simulink model "model_sim_CHB5_36_new_temp"  (R2020a)
settings: Solver=FixedStepAuto  StartTime=0.0  StopTime=5  RelTol=1e-3
InitFcn:
  | sysinit
values from neighbouring files (symbols this model uses):
  C = 0.03    [sysinit.m]
  C_f = 0.625e-6    (= 6.25e-07)    [sysinit.m]
  f = 50    [sysinit.m]
  f_switch = 500    [sysinit.m]
  L = 0.004    [sysinit.m]
  L_f = 3e-6    (= 3e-06)    [sysinit.m]
  R = 1.2    [sysinit.m]
  R_f = 1.5    [sysinit.m]
  Rth_h = 7.5e-3    (= 0.0075)    [Device_Parameter.m]
  Rth_h_tau = 0.5    [Device_Parameter.m]
  st = 5e-7    (= 5e-07)    [sysinit.m]
  temp_init = 40    [sysinit.m]
  Ts = 1e-6    (= 1e-06)    [sysinit.m]
  Ts2 = 0.5E-3    (= 0.0005)    [sysinit.m]
  Udc = 2500    [sysinit.m]
undefined symbols (not defined in the file or in its folder): DIODE_204520, DIODE_344520, DIODE_D1031SH, DIODE_D1331SH, IGCT_364520_36, IGCT_364521_36, IGCT_654522_6, magnitude, Ts1
libraries: powerlib x278, powerlib_meascontrol x84, simulink x9
(part 4 of 5)

== system model_sim_CHB5_36_new_temp/Subsystem3/DIODE/DIODE_204520/Subsystem5/Subsystem1 ==
  note: 用于判断D1关断时刻，电流为负时，T3开通就意味着D1关断
  In1 : Inport
  In2 : Inport  Port=2
  Abs1 : Abs
  Add : Sum
  Constant1 : Constant  Value=0
  Constant2 : Constant  Value=0
  Gain1 : Gain  Gain=Udc/DIODE.Vdc
  Gain2 : Gain  Gain=DIODE.Err/DIODE.IFQ
  Gain3 : Gain  Gain=1/Ts2
  Gain4 : Gain
  Logical Operator2 : Logic  Operator=NOT  AllPortsSameDT=off  OutDataTypeStr=boolean
  Logical Operator3 : Logic  AllPortsSameDT=off  OutDataTypeStr=boolean
  Logical Operator4 : Logic  AllPortsSameDT=off  OutDataTypeStr=boolean
  Logical Operator5 : Logic  Operator=NOT  AllPortsSameDT=off  OutDataTypeStr=boolean
  Pulse Generator : DiscretePulseGenerator  PulseType=Time based  Period=Ts2  PulseWidth=5
  Saturation : Saturate  UpperLimit=5500  LowerLimit=0
  Saturation1 : Saturate  UpperLimit=100  LowerLimit=0
  Switch2 : Switch  Criteria=u2 > Threshold
  Switch3 : Switch  Criteria=u2 > Threshold
  Switch4 : Switch  Criteria=u2 > Threshold
  Unit Delay{,1..3} (4 alike) : UnitDelay  SampleTime=Ts1  HasFrameUpgradeWarning=on
  Out1 : Outport  VectorParamsAs1DForOutWhenUnconnected=off
  wires:
  Gain2/1 -> Saturation1/1
  Saturation/1 -> Gain2/1
  Saturation1/1 -> Switch2/1
  Gain4/1 -> Saturation/1
  Unit Delay/1 -> Logical Operator2/1
  Add/1 -> Unit Delay1/1
  In1/1 -> Gain4/1
  Gain3/1 -> Out1/1
  Unit Delay1/1 -> Switch4/1, Switch3/3
  Logical Operator4/1 -> Switch3/2, Switch4/2
  Logical Operator5/1 -> Logical Operator4/2
  Unit Delay3/1 -> Logical Operator5/1
  Unit Delay2/1 -> Switch4/3
  Switch4/1 -> Gain3/1, Unit Delay2/1
  Pulse Generator/1 -> Logical Operator4/1, Unit Delay3/1
  Constant1/1 -> Switch3/1
  Switch3/1 -> Add/2
  Constant2/1 -> Switch2/3
  Logical Operator3/1 -> Switch2/2
  Logical Operator2/1 -> Logical Operator3/2
  In2/1 -> Unit Delay/1, Logical Operator3/1
  Gain1/1 -> Abs1/1
  Switch2/1 -> Gain1/1
  Abs1/1 -> Add/1

== system model_sim_CHB5_36_new_temp/Subsystem3/DIODE/DIODE_204520/Subsystem5/Subsystem2 ==
  note: 器件手册热阻：壳到结
  note: 散热器热阻：水到壳
  In1 : Inport
  In2 : Inport  Port=2
  Add3 : Sum
  Add4 : Sum  Inputs=4
  Add5 : Sum  Inputs=+++
  Constant : Constant  Value=temp_init
  Discrete Filter1 : DiscreteFilter  Numerator=[Ts2/DIODE_344520.Rth_jc1_dou_tau]  Denominator=[1 (Ts2/DIODE_344520.Rth_jc1_dou_tau)-1]  SampleTime=Ts2
  Discrete Filter2 : DiscreteFilter  Numerator=[Ts2/DIODE_344520.Rth_jc2_dou_tau]  Denominator=[1 (Ts2/DIODE_344520.Rth_jc2_dou_tau)-1]  SampleTime=Ts2
  Discrete Filter3 : DiscreteFilter  Numerator=[Ts2/DIODE_344520.Rth_jc3_dou_tau]  Denominator=[1 (Ts2/DIODE_344520.Rth_jc3_dou_tau)-1]  SampleTime=Ts2
  Discrete Filter5 : DiscreteFilter  Numerator=[Ts2/DIODE_344520.Rth_ch_dou_tau]  Denominator=[1 (Ts2/DIODE_344520.Rth_ch_dou_tau)-1]  SampleTime=Ts2
  Discrete Filter9 : DiscreteFilter  Numerator=[Ts2/Rth_h_tau]  Denominator=[1 (Ts2/Rth_h_tau)-1]  SampleTime=Ts2
  Gain1 : Gain  Gain=DIODE_344520.Rth_jc1_dou
  Gain2 : Gain  Gain=DIODE_344520.Rth_jc2_dou
  Gain3 : Gain  Gain=DIODE_344520.Rth_jc3_dou
  Gain5 : Gain  Gain=DIODE_344520.Rth_ch_dou
  Gain9 : Gain  Gain=Rth_h
  Out1 : Outport  VectorParamsAs1DForOutWhenUnconnected=off
  wires:
  Discrete Filter9/1 -> Add5/1
  Gain9/1 -> Discrete Filter9/1
  Add3/1 -> Gain2/1, Gain1/1, Gain9/1, Gain5/1, Gain3/1
  Discrete Filter3/1 -> Add4/4
  Gain3/1 -> Discrete Filter3/1
  Discrete Filter5/1 -> Add4/1
  Gain5/1 -> Discrete Filter5/1
  Discrete Filter1/1 -> Add4/2
  Add5/1 -> Out1/1
  Gain1/1 -> Discrete Filter1/1
  Constant/1 -> Add5/3
  In2/1 -> Add3/2
  Add4/1 -> Add5/2
  Discrete Filter2/1 -> Add4/3
  Gain2/1 -> Discrete Filter2/1
  In1/1 -> Add3/1

== system model_sim_CHB5_36_new_temp/Subsystem3/DIODE/DIODE_204520/Subsystem5/Subsystem29 ==
  note: 用于判断D1关断时刻，电流为负时，T3开通就意味着D1关断
  In1 : Inport
  In2 : Inport  Port=2
  Abs1 : Abs
  Add : Sum
  Constant1 : Constant  Value=0
  Constant2 : Constant  Value=0
  Gain1 : Gain  Gain=Udc/DIODE.Vdc
  Gain2 : Gain  Gain=DIODE.Err/DIODE.IFQ
  Gain3 : Gain  Gain=1/Ts2
  Gain4 : Gain
  Logical Operator2 : Logic  Operator=NOT  AllPortsSameDT=off  OutDataTypeStr=boolean
  Logical Operator3 : Logic  AllPortsSameDT=off  OutDataTypeStr=boolean
  Logical Operator4 : Logic  AllPortsSameDT=off  OutDataTypeStr=boolean
  Logical Operator5 : Logic  Operator=NOT  AllPortsSameDT=off  OutDataTypeStr=boolean
  Pulse Generator : DiscretePulseGenerator  PulseType=Time based  Period=Ts2  PulseWidth=5
  Saturation : Saturate  UpperLimit=5500  LowerLimit=0
  Saturation1 : Saturate  UpperLimit=100  LowerLimit=0
  Switch2 : Switch  Criteria=u2 > Threshold
  Switch3 : Switch  Criteria=u2 > Threshold
  Switch4 : Switch  Criteria=u2 > Threshold
  Unit Delay{,1..3} (4 alike) : UnitDelay  SampleTime=Ts1  HasFrameUpgradeWarning=on
  Out1 : Outport  VectorParamsAs1DForOutWhenUnconnected=off
  wires:
  Gain2/1 -> Saturation1/1
  Saturation/1 -> Gain2/1
  Saturation1/1 -> Switch2/1
  Gain4/1 -> Saturation/1
  Unit Delay/1 -> Logical Operator2/1
  Add/1 -> Unit Delay1/1
  In1/1 -> Gain4/1
  Gain3/1 -> Out1/1
  Unit Delay1/1 -> Switch4/1, Switch3/3
  Logical Operator4/1 -> Switch3/2, Switch4/2
  Logical Operator5/1 -> Logical Operator4/2
  Unit Delay3/1 -> Logical Operator5/1
  Unit Delay2/1 -> Switch4/3
  Switch4/1 -> Gain3/1, Unit Delay2/1
  Pulse Generator/1 -> Logical Operator4/1, Unit Delay3/1
  Constant1/1 -> Switch3/1
  Switch3/1 -> Add/2
  Constant2/1 -> Switch2/3
  Logical Operator3/1 -> Switch2/2
  Logical Operator2/1 -> Logical Operator3/2
  In2/1 -> Unit Delay/1, Logical Operator3/1
  Gain1/1 -> Abs1/1
  Switch2/1 -> Gain1/1
  Abs1/1 -> Add/1

== system model_sim_CHB5_36_new_temp/Subsystem3/DIODE/DIODE_204520/Subsystem5/Subsystem4 ==
  In1 : Inport
  Gain44 : Gain  Gain=DIODE.rF
  Gain45 : Gain  Gain=DIODE.VF0
  Math Function9 : Math  Operator=magnitude^2  SignedPower=on  SaturateOnIntegerOverflow=on
  Mean79 : powerlib_meascontrol/Measurements/Mean  Freq=2000  Vinit=0  Ts=Ts1
  RMS9 : powerlib_meascontrol/Measurements/RMS  TrueRMS=on  Freq=2000  RMSInit=0  Ts=Ts1
  Out1 : Outport
  Out2 : Outport  Port=2
  wires:
  RMS9/1 -> Math Function9/1
  Gain44/1 -> Out1/1
  Mean79/1 -> Gain45/1
  Math Function9/1 -> Gain44/1
  In1/1 -> Mean79/1, RMS9/1
  Gain45/1 -> Out2/1

== system model_sim_CHB5_36_new_temp/Subsystem3/DIODE/DIODE_204520/Subsystem5/Subsystem53 ==
  note: 器件手册热阻：壳到结
  note: 散热器热阻：水到壳
  In1 : Inport
  In2 : Inport  Port=2
  Add3 : Sum
  Add4 : Sum  Inputs=4
  Add5 : Sum  Inputs=+++
  Constant : Constant  Value=temp_init
  Discrete Filter1 : DiscreteFilter  Numerator=[Ts2/DIODE_344520.Rth_jc1_dou_tau]  Denominator=[1 (Ts2/DIODE_344520.Rth_jc1_dou_tau)-1]  SampleTime=Ts2
  Discrete Filter2 : DiscreteFilter  Numerator=[Ts2/DIODE_344520.Rth_jc2_dou_tau]  Denominator=[1 (Ts2/DIODE_344520.Rth_jc2_dou_tau)-1]  SampleTime=Ts2
  Discrete Filter3 : DiscreteFilter  Numerator=[Ts2/DIODE_344520.Rth_jc3_dou_tau]  Denominator=[1 (Ts2/DIODE_344520.Rth_jc3_dou_tau)-1]  SampleTime=Ts2
  Discrete Filter5 : DiscreteFilter  Numerator=[Ts2/DIODE_344520.Rth_ch_dou_tau]  Denominator=[1 (Ts2/DIODE_344520.Rth_ch_dou_tau)-1]  SampleTime=Ts2
  Discrete Filter9 : DiscreteFilter  Numerator=[Ts2/Rth_h_tau]  Denominator=[1 (Ts2/Rth_h_tau)-1]  SampleTime=Ts2
  Gain1 : Gain  Gain=DIODE_344520.Rth_jc1_dou
  Gain2 : Gain  Gain=DIODE_344520.Rth_jc2_dou
  Gain3 : Gain  Gain=DIODE_344520.Rth_jc3_dou
  Gain5 : Gain  Gain=DIODE_344520.Rth_ch_dou
  Gain9 : Gain  Gain=Rth_h
  Out1 : Outport  VectorParamsAs1DForOutWhenUnconnected=off
  wires:
  Discrete Filter9/1 -> Add5/1
  Gain9/1 -> Discrete Filter9/1
  Add3/1 -> Gain2/1, Gain1/1, Gain9/1, Gain5/1, Gain3/1
  Discrete Filter3/1 -> Add4/4
  Gain3/1 -> Discrete Filter3/1
  Discrete Filter5/1 -> Add4/1
  Gain5/1 -> Discrete Filter5/1
  Discrete Filter1/1 -> Add4/2
  Add5/1 -> Out1/1
  Gain1/1 -> Discrete Filter1/1
  Constant/1 -> Add5/3
  In2/1 -> Add3/2
  Add4/1 -> Add5/2
  Discrete Filter2/1 -> Add4/3
  Gain2/1 -> Discrete Filter2/1
  In1/1 -> Add3/1

== system model_sim_CHB5_36_new_temp/Subsystem3/DIODE/DIODE_344520/Subsystem5/Subsystem ==
  In1 : Inport
  Gain44 : Gain  Gain=DIODE.rF
  Gain45 : Gain  Gain=DIODE.VF0
  Math Function9 : Math  Operator=magnitude^2  SignedPower=on  SaturateOnIntegerOverflow=on
  Mean79 : powerlib_meascontrol/Measurements/Mean  Freq=2000  Vinit=0  Ts=Ts
  RMS9 : powerlib_meascontrol/Measurements/RMS  TrueRMS=on  Freq=2000  RMSInit=0  Ts=Ts1
  Out1 : Outport
  Out2 : Outport  Port=2
  wires:
  Gain45/1 -> Out2/1
  In1/1 -> RMS9/1, Mean79/1
  Math Function9/1 -> Gain44/1
  Mean79/1 -> Gain45/1
  Gain44/1 -> Out1/1
  RMS9/1 -> Math Function9/1

== system model_sim_CHB5_36_new_temp/Subsystem3/DIODE/DIODE_344520/Subsystem5/Subsystem1 ==
  note: 用于判断D1关断时刻，电流为负时，T3开通就意味着D1关断
  In1 : Inport
  In2 : Inport  Port=2
  Abs1 : Abs
  Add : Sum
  Constant1 : Constant  Value=0
  Constant2 : Constant  Value=0
  Gain1 : Gain  Gain=Udc/DIODE.Vdc
  Gain2 : Gain  Gain=DIODE.Err/DIODE.IFQ
  Gain3 : Gain  Gain=1/Ts2
  Gain4 : Gain
  Logical Operator2 : Logic  Operator=NOT  AllPortsSameDT=off  OutDataTypeStr=boolean
  Logical Operator3 : Logic  AllPortsSameDT=off  OutDataTypeStr=boolean
  Logical Operator4 : Logic  AllPortsSameDT=off  OutDataTypeStr=boolean
  Logical Operator5 : Logic  Operator=NOT  AllPortsSameDT=off  OutDataTypeStr=boolean
  Pulse Generator : DiscretePulseGenerator  PulseType=Time based  Period=Ts2  PulseWidth=5
  Saturation : Saturate  UpperLimit=5500  LowerLimit=0
  Saturation1 : Saturate  UpperLimit=100  LowerLimit=0
  Switch2 : Switch  Criteria=u2 > Threshold
  Switch3 : Switch  Criteria=u2 > Threshold
  Switch4 : Switch  Criteria=u2 > Threshold
  Unit Delay{,1..3} (4 alike) : UnitDelay  SampleTime=Ts1  HasFrameUpgradeWarning=on
  Out1 : Outport  VectorParamsAs1DForOutWhenUnconnected=off
  wires:
  Abs1/1 -> Add/1
  Switch2/1 -> Gain1/1
  Gain1/1 -> Abs1/1
  In2/1 -> Logical Operator3/1, Unit Delay/1
  Logical Operator2/1 -> Logical Operator3/2
  Logical Operator3/1 -> Switch2/2
  Constant2/1 -> Switch2/3
  Switch3/1 -> Add/2
  Constant1/1 -> Switch3/1
  Pulse Generator/1 -> Unit Delay3/1, Logical Operator4/1
  Switch4/1 -> Unit Delay2/1, Gain3/1
  Unit Delay2/1 -> Switch4/3
  Unit Delay3/1 -> Logical Operator5/1
  Logical Operator5/1 -> Logical Operator4/2
  Logical Operator4/1 -> Switch4/2, Switch3/2
  Unit Delay1/1 -> Switch3/3, Switch4/1
  Gain3/1 -> Out1/1
  In1/1 -> Gain4/1
  Add/1 -> Unit Delay1/1
  Unit Delay/1 -> Logical Operator2/1
  Gain4/1 -> Saturation/1
  Saturation1/1 -> Switch2/1
  Saturation/1 -> Gain2/1
  Gain2/1 -> Saturation1/1

== system model_sim_CHB5_36_new_temp/Subsystem3/DIODE/DIODE_344520/Subsystem5/Subsystem2 ==
  note: 散热器热阻：水到壳
  note: 器件手册热阻：壳到结
  In1 : Inport
  In2 : Inport  Port=2
  Add3 : Sum
  Add4 : Sum  Inputs=4
  Add5 : Sum  Inputs=+++
  Constant : Constant  Value=temp_init
  Discrete Filter1 : DiscreteFilter  Numerator=[Ts2/DIODE_344520.Rth_jc1_dou_tau]  Denominator=[1 (Ts2/DIODE_344520.Rth_jc1_dou_tau)-1]  SampleTime=Ts2
  Discrete Filter2 : DiscreteFilter  Numerator=[Ts2/DIODE_344520.Rth_jc2_dou_tau]  Denominator=[1 (Ts2/DIODE_344520.Rth_jc2_dou_tau)-1]  SampleTime=Ts2
  Discrete Filter3 : DiscreteFilter  Numerator=[Ts2/DIODE_344520.Rth_jc3_dou_tau]  Denominator=[1 (Ts2/DIODE_344520.Rth_jc3_dou_tau)-1]  SampleTime=Ts2
  Discrete Filter5 : DiscreteFilter  Numerator=[Ts2/DIODE_344520.Rth_ch_dou_tau]  Denominator=[1 (Ts2/DIODE_344520.Rth_ch_dou_tau)-1]  SampleTime=Ts2
  Discrete Filter9 : DiscreteFilter  Numerator=[Ts2/Rth_h_tau]  Denominator=[1 (Ts2/Rth_h_tau)-1]  SampleTime=Ts2
  Gain1 : Gain  Gain=DIODE_344520.Rth_jc1_dou
  Gain2 : Gain  Gain=DIODE_344520.Rth_jc2_dou
  Gain3 : Gain  Gain=DIODE_344520.Rth_jc3_dou
  Gain5 : Gain  Gain=DIODE_344520.Rth_ch_dou
  Gain9 : Gain  Gain=Rth_h
  Out1 : Outport  VectorParamsAs1DForOutWhenUnconnected=off
  wires:
  In1/1 -> Add3/1
  Gain2/1 -> Discrete Filter2/1
  Discrete Filter2/1 -> Add4/3
  Add4/1 -> Add5/2
  In2/1 -> Add3/2
  Constant/1 -> Add5/3
  Gain1/1 -> Discrete Filter1/1
  Add5/1 -> Out1/1
  Discrete Filter1/1 -> Add4/2
  Gain5/1 -> Discrete Filter5/1
  Discrete Filter5/1 -> Add4/1
  Gain3/1 -> Discrete Filter3/1
  Discrete Filter3/1 -> Add4/4
  Add3/1 -> Gain3/1, Gain5/1, Gain9/1, Gain1/1, Gain2/1
  Gain9/1 -> Discrete Filter9/1
  Discrete Filter9/1 -> Add5/1

== system model_sim_CHB5_36_new_temp/Subsystem3/DIODE/DIODE_344520/Subsystem5/Subsystem29 ==
  note: 用于判断D1关断时刻，电流为负时，T3开通就意味着D1关断
  In1 : Inport
  In2 : Inport  Port=2
  Abs1 : Abs
  Add : Sum
  Constant1 : Constant  Value=0
  Constant2 : Constant  Value=0
  Gain1 : Gain  Gain=Udc/DIODE.Vdc
  Gain2 : Gain  Gain=DIODE.Err/DIODE.IFQ
  Gain3 : Gain  Gain=1/Ts2
  Gain4 : Gain
  Logical Operator2 : Logic  Operator=NOT  AllPortsSameDT=off  OutDataTypeStr=boolean
  Logical Operator3 : Logic  AllPortsSameDT=off  OutDataTypeStr=boolean
  Logical Operator4 : Logic  AllPortsSameDT=off  OutDataTypeStr=boolean
  Logical Operator5 : Logic  Operator=NOT  AllPortsSameDT=off  OutDataTypeStr=boolean
  Pulse Generator : DiscretePulseGenerator  PulseType=Time based  Period=Ts2  PulseWidth=5
  Saturation : Saturate  UpperLimit=5500  LowerLimit=0
  Saturation1 : Saturate  UpperLimit=100  LowerLimit=0
  Switch2 : Switch  Criteria=u2 > Threshold
  Switch3 : Switch  Criteria=u2 > Threshold
  Switch4 : Switch  Criteria=u2 > Threshold
  Unit Delay{,1..3} (4 alike) : UnitDelay  SampleTime=Ts1  HasFrameUpgradeWarning=on
  Out1 : Outport  VectorParamsAs1DForOutWhenUnconnected=off
  wires:
  Abs1/1 -> Add/1
  Switch2/1 -> Gain1/1
  Gain1/1 -> Abs1/1
  In2/1 -> Logical Operator3/1, Unit Delay/1
  Logical Operator2/1 -> Logical Operator3/2
  Logical Operator3/1 -> Switch2/2
  Constant2/1 -> Switch2/3
  Switch3/1 -> Add/2
  Constant1/1 -> Switch3/1
  Pulse Generator/1 -> Unit Delay3/1, Logical Operator4/1
  Switch4/1 -> Unit Delay2/1, Gain3/1
  Unit Delay2/1 -> Switch4/3
  Unit Delay3/1 -> Logical Operator5/1
  Logical Operator5/1 -> Logical Operator4/2
  Logical Operator4/1 -> Switch4/2, Switch3/2
  Unit Delay1/1 -> Switch3/3, Switch4/1
  Gain3/1 -> Out1/1
  In1/1 -> Gain4/1
  Add/1 -> Unit Delay1/1
  Unit Delay/1 -> Logical Operator2/1
  Gain4/1 -> Saturation/1
  Saturation1/1 -> Switch2/1
  Saturation/1 -> Gain2/1
  Gain2/1 -> Saturation1/1

== system model_sim_CHB5_36_new_temp/Subsystem3/DIODE/DIODE_344520/Subsystem5/Subsystem4 ==
  In1 : Inport
  Gain44 : Gain  Gain=DIODE.rF
  Gain45 : Gain  Gain=DIODE.VF0
  Math Function9 : Math  Operator=magnitude^2  SignedPower=on  SaturateOnIntegerOverflow=on
  Mean79 : powerlib_meascontrol/Measurements/Mean  Freq=2000  Vinit=0  Ts=Ts1
  RMS9 : powerlib_meascontrol/Measurements/RMS  TrueRMS=on  Freq=2000  RMSInit=0  Ts=Ts1
  Out1 : Outport
  Out2 : Outport  Port=2
  wires:
  Gain45/1 -> Out2/1
  In1/1 -> RMS9/1, Mean79/1
  Math Function9/1 -> Gain44/1
  Mean79/1 -> Gain45/1
  Gain44/1 -> Out1/1
  RMS9/1 -> Math Function9/1

== system model_sim_CHB5_36_new_temp/Subsystem3/DIODE/DIODE_344520/Subsystem5/Subsystem53 ==
  note: 散热器热阻：水到壳
  note: 器件手册热阻：壳到结
  In1 : Inport
  In2 : Inport  Port=2
  Add3 : Sum
  Add4 : Sum  Inputs=4
  Add5 : Sum  Inputs=+++
  Constant : Constant  Value=temp_init
  Discrete Filter1 : DiscreteFilter  Numerator=[Ts2/DIODE_344520.Rth_jc1_dou_tau]  Denominator=[1 (Ts2/DIODE_344520.Rth_jc1_dou_tau)-1]  SampleTime=Ts2
  Discrete Filter2 : DiscreteFilter  Numerator=[Ts2/DIODE_344520.Rth_jc2_dou_tau]  Denominator=[1 (Ts2/DIODE_344520.Rth_jc2_dou_tau)-1]  SampleTime=Ts2
  Discrete Filter3 : DiscreteFilter  Numerator=[Ts2/DIODE_344520.Rth_jc3_dou_tau]  Denominator=[1 (Ts2/DIODE_344520.Rth_jc3_dou_tau)-1]  SampleTime=Ts2
  Discrete Filter5 : DiscreteFilter  Numerator=[Ts2/DIODE_344520.Rth_ch_dou_tau]  Denominator=[1 (Ts2/DIODE_344520.Rth_ch_dou_tau)-1]  SampleTime=Ts2
  Discrete Filter9 : DiscreteFilter  Numerator=[Ts2/Rth_h_tau]  Denominator=[1 (Ts2/Rth_h_tau)-1]  SampleTime=Ts2
  Gain1 : Gain  Gain=DIODE_344520.Rth_jc1_dou
  Gain2 : Gain  Gain=DIODE_344520.Rth_jc2_dou
  Gain3 : Gain  Gain=DIODE_344520.Rth_jc3_dou
  Gain5 : Gain  Gain=DIODE_344520.Rth_ch_dou
  Gain9 : Gain  Gain=Rth_h
  Out1 : Outport  VectorParamsAs1DForOutWhenUnconnected=off
  wires:
  In1/1 -> Add3/1
  Gain2/1 -> Discrete Filter2/1
  Discrete Filter2/1 -> Add4/3
  Add4/1 -> Add5/2
  In2/1 -> Add3/2
  Constant/1 -> Add5/3
  Gain1/1 -> Discrete Filter1/1
  Add5/1 -> Out1/1
  Discrete Filter1/1 -> Add4/2
  Gain5/1 -> Discrete Filter5/1
  Discrete Filter5/1 -> Add4/1
  Gain3/1 -> Discrete Filter3/1
  Discrete Filter3/1 -> Add4/4
  Add3/1 -> Gain3/1, Gain5/1, Gain9/1, Gain1/1, Gain2/1
  Gain9/1 -> Discrete Filter9/1
  Discrete Filter9/1 -> Add5/1

== system model_sim_CHB5_36_new_temp/Subsystem3/DIODE/DIODE_D1031SH/Subsystem5/Subsystem ==
  In1 : Inport
  Gain44 : Gain  Gain=DIODE.rF
  Gain45 : Gain  Gain=DIODE.VF0
  Math Function9 : Math  Operator=magnitude^2  SignedPower=on  SaturateOnIntegerOverflow=on
  Mean79 : powerlib_meascontrol/Measurements/Mean  Freq=2000  Vinit=0  Ts=Ts1
  RMS9 : powerlib_meascontrol/Measurements/RMS  TrueRMS=on  Freq=2000  RMSInit=0  Ts=Ts1
  Out1 : Outport
  Out2 : Outport  Port=2
  wires:
  RMS9/1 -> Math Function9/1
  Gain44/1 -> Out1/1
  Mean79/1 -> Gain45/1
  Math Function9/1 -> Gain44/1
  In1/1 -> Mean79/1, RMS9/1
  Gain45/1 -> Out2/1

== system model_sim_CHB5_36_new_temp/Subsystem3/DIODE/DIODE_D1031SH/Subsystem5/Subsystem1 ==
  note: 用于判断D1关断时刻，电流为负时，T3开通就意味着D1关断
  In1 : Inport
  In2 : Inport  Port=2
  Abs1 : Abs
  Add : Sum
  Constant1 : Constant  Value=0
  Constant2 : Constant  Value=0
  Gain1 : Gain  Gain=Udc/DIODE.Vdc
  Gain2 : Gain  Gain=DIODE.Err/DIODE.IFQ
  Gain3 : Gain  Gain=1/Ts2
  Gain4 : Gain
  Logical Operator2 : Logic  Operator=NOT  AllPortsSameDT=off  OutDataTypeStr=boolean
  Logical Operator3 : Logic  AllPortsSameDT=off  OutDataTypeStr=boolean
  Logical Operator4 : Logic  AllPortsSameDT=off  OutDataTypeStr=boolean
  Logical Operator5 : Logic  Operator=NOT  AllPortsSameDT=off  OutDataTypeStr=boolean
  Pulse Generator : DiscretePulseGenerator  PulseType=Time based  Period=Ts2  PulseWidth=5
  Saturation : Saturate  UpperLimit=5500  LowerLimit=0
  Saturation1 : Saturate  UpperLimit=100  LowerLimit=0
  Switch2 : Switch  Criteria=u2 > Threshold
  Switch3 : Switch  Criteria=u2 > Threshold
  Switch4 : Switch  Criteria=u2 > Threshold
  Unit Delay{,1..3} (4 alike) : UnitDelay  SampleTime=Ts1  HasFrameUpgradeWarning=on
  Out1 : Outport  VectorParamsAs1DForOutWhenUnconnected=off
  wires:
  Gain2/1 -> Saturation1/1
  Saturation/1 -> Gain2/1
  Saturation1/1 -> Switch2/1
  Gain4/1 -> Saturation/1
  Unit Delay/1 -> Logical Operator2/1
  Add/1 -> Unit Delay1/1
  In1/1 -> Gain4/1
  Gain3/1 -> Out1/1
  Unit Delay1/1 -> Switch4/1, Switch3/3
  Logical Operator4/1 -> Switch3/2, Switch4/2
  Logical Operator5/1 -> Logical Operator4/2
  Unit Delay3/1 -> Logical Operator5/1
  Unit Delay2/1 -> Switch4/3
  Switch4/1 -> Gain3/1, Unit Delay2/1
  Pulse Generator/1 -> Logical Operator4/1, Unit Delay3/1
  Constant1/1 -> Switch3/1
  Switch3/1 -> Add/2
  Constant2/1 -> Switch2/3
  Logical Operator3/1 -> Switch2/2
  Logical Operator2/1 -> Logical Operator3/2
  In2/1 -> Unit Delay/1, Logical Operator3/1
  Gain1/1 -> Abs1/1
  Switch2/1 -> Gain1/1
  Abs1/1 -> Add/1

== system model_sim_CHB5_36_new_temp/Subsystem3/DIODE/DIODE_D1031SH/Subsystem5/Subsystem2 ==
  note: 器件手册热阻：壳到结
  note: 散热器热阻：水到壳
  In1 : Inport
  In2 : Inport  Port=2
  Add3 : Sum
  Add4 : Sum  Inputs=4
  Add5 : Sum  Inputs=+++
  Constant : Constant  Value=temp_init
  Discrete Filter1 : DiscreteFilter  Numerator=[Ts2/DIODE_344520.Rth_jc1_dou_tau]  Denominator=[1 (Ts2/DIODE_344520.Rth_jc1_dou_tau)-1]  SampleTime=Ts2
  Discrete Filter2 : DiscreteFilter  Numerator=[Ts2/DIODE_344520.Rth_jc2_dou_tau]  Denominator=[1 (Ts2/DIODE_344520.Rth_jc2_dou_tau)-1]  SampleTime=Ts2
  Discrete Filter3 : DiscreteFilter  Numerator=[Ts2/DIODE_344520.Rth_jc3_dou_tau]  Denominator=[1 (Ts2/DIODE_344520.Rth_jc3_dou_tau)-1]  SampleTime=Ts2
  Discrete Filter5 : DiscreteFilter  Numerator=[Ts2/DIODE_344520.Rth_ch_dou_tau]  Denominator=[1 (Ts2/DIODE_344520.Rth_ch_dou_tau)-1]  SampleTime=Ts2
  Discrete Filter9 : DiscreteFilter  Numerator=[Ts2/Rth_h_tau]  Denominator=[1 (Ts2/Rth_h_tau)-1]  SampleTime=Ts2
  Gain1 : Gain  Gain=DIODE_344520.Rth_jc1_dou
  Gain2 : Gain  Gain=DIODE_344520.Rth_jc2_dou
  Gain3 : Gain  Gain=DIODE_344520.Rth_jc3_dou
  Gain5 : Gain  Gain=DIODE_344520.Rth_ch_dou
  Gain9 : Gain  Gain=Rth_h
  Out1 : Outport  VectorParamsAs1DForOutWhenUnconnected=off
  wires:
  Discrete Filter9/1 -> Add5/1
  Gain9/1 -> Discrete Filter9/1
  Add3/1 -> Gain2/1, Gain1/1, Gain9/1, Gain5/1, Gain3/1
  Discrete Filter3/1 -> Add4/4
  Gain3/1 -> Discrete Filter3/1
  Discrete Filter5/1 -> Add4/1
  Gain5/1 -> Discrete Filter5/1
  Discrete Filter1/1 -> Add4/2
  Add5/1 -> Out1/1
  Gain1/1 -> Discrete Filter1/1
  Constant/1 -> Add5/3
  In2/1 -> Add3/2
  Add4/1 -> Add5/2
  Discrete Filter2/1 -> Add4/3
  Gain2/1 -> Discrete Filter2/1
  In1/1 -> Add3/1

== system model_sim_CHB5_36_new_temp/Subsystem3/DIODE/DIODE_D1031SH/Subsystem5/Subsystem29 ==
  note: 用于判断D1关断时刻，电流为负时，T3开通就意味着D1关断
  In1 : Inport
  In2 : Inport  Port=2
  Abs1 : Abs
  Add : Sum
  Constant1 : Constant  Value=0
  Constant2 : Constant  Value=0
  Gain1 : Gain  Gain=Udc/DIODE.Vdc
  Gain2 : Gain  Gain=DIODE.Err/DIODE.IFQ
  Gain3 : Gain  Gain=1/Ts2
  Gain4 : Gain
  Logical Operator2 : Logic  Operator=NOT  AllPortsSameDT=off  OutDataTypeStr=boolean
  Logical Operator3 : Logic  AllPortsSameDT=off  OutDataTypeStr=boolean
  Logical Operator4 : Logic  AllPortsSameDT=off  OutDataTypeStr=boolean
  Logical Operator5 : Logic  Operator=NOT  AllPortsSameDT=off  OutDataTypeStr=boolean
  Pulse Generator : DiscretePulseGenerator  PulseType=Time based  Period=Ts2  PulseWidth=5
  Saturation : Saturate  UpperLimit=5500  LowerLimit=0
  Saturation1 : Saturate  UpperLimit=100  LowerLimit=0
  Switch2 : Switch  Criteria=u2 > Threshold
  Switch3 : Switch  Criteria=u2 > Threshold
  Switch4 : Switch  Criteria=u2 > Threshold
  Unit Delay{,1..3} (4 alike) : UnitDelay  SampleTime=Ts1  HasFrameUpgradeWarning=on
  Out1 : Outport  VectorParamsAs1DForOutWhenUnconnected=off
  wires:
  Gain2/1 -> Saturation1/1
  Saturation/1 -> Gain2/1
  Saturation1/1 -> Switch2/1
  Gain4/1 -> Saturation/1
  Unit Delay/1 -> Logical Operator2/1
  Add/1 -> Unit Delay1/1
  In1/1 -> Gain4/1
  Gain3/1 -> Out1/1
  Unit Delay1/1 -> Switch4/1, Switch3/3
  Logical Operator4/1 -> Switch3/2, Switch4/2
  Logical Operator5/1 -> Logical Operator4/2
  Unit Delay3/1 -> Logical Operator5/1
  Unit Delay2/1 -> Switch4/3
  Switch4/1 -> Gain3/1, Unit Delay2/1
  Pulse Generator/1 -> Logical Operator4/1, Unit Delay3/1
  Constant1/1 -> Switch3/1
  Switch3/1 -> Add/2
  Constant2/1 -> Switch2/3
  Logical Operator3/1 -> Switch2/2
  Logical Operator2/1 -> Logical Operator3/2
  In2/1 -> Unit Delay/1, Logical Operator3/1
  Gain1/1 -> Abs1/1
  Switch2/1 -> Gain1/1
  Abs1/1 -> Add/1

== system model_sim_CHB5_36_new_temp/Subsystem3/DIODE/DIODE_D1031SH/Subsystem5/Subsystem4 ==
  In1 : Inport
  Gain44 : Gain  Gain=DIODE.rF
  Gain45 : Gain  Gain=DIODE.VF0
  Math Function9 : Math  Operator=magnitude^2  SignedPower=on  SaturateOnIntegerOverflow=on
  Mean79 : powerlib_meascontrol/Measurements/Mean  Freq=2000  Vinit=0  Ts=Ts1
  RMS9 : powerlib_meascontrol/Measurements/RMS  TrueRMS=on  Freq=2000  RMSInit=0  Ts=Ts1
  Out1 : Outport
  Out2 : Outport  Port=2
  wires:
  RMS9/1 -> Math Function9/1
  Gain44/1 -> Out1/1
  Mean79/1 -> Gain45/1
  Math Function9/1 -> Gain44/1
  In1/1 -> Mean79/1, RMS9/1
  Gain45/1 -> Out2/1

== system model_sim_CHB5_36_new_temp/Subsystem3/DIODE/DIODE_D1031SH/Subsystem5/Subsystem53 ==
  note: 器件手册热阻：壳到结
  note: 散热器热阻：水到壳
  In1 : Inport
  In2 : Inport  Port=2
  Add3 : Sum
  Add4 : Sum  Inputs=4
  Add5 : Sum  Inputs=+++
  Constant : Constant  Value=temp_init
  Discrete Filter1 : DiscreteFilter  Numerator=[Ts2/DIODE_344520.Rth_jc1_dou_tau]  Denominator=[1 (Ts2/DIODE_344520.Rth_jc1_dou_tau)-1]  SampleTime=Ts2
  Discrete Filter2 : DiscreteFilter  Numerator=[Ts2/DIODE_344520.Rth_jc2_dou_tau]  Denominator=[1 (Ts2/DIODE_344520.Rth_jc2_dou_tau)-1]  SampleTime=Ts2
  Discrete Filter3 : DiscreteFilter  Numerator=[Ts2/DIODE_344520.Rth_jc3_dou_tau]  Denominator=[1 (Ts2/DIODE_344520.Rth_jc3_dou_tau)-1]  SampleTime=Ts2
  Discrete Filter5 : DiscreteFilter  Numerator=[Ts2/DIODE_344520.Rth_ch_dou_tau]  Denominator=[1 (Ts2/DIODE_344520.Rth_ch_dou_tau)-1]  SampleTime=Ts2
  Discrete Filter9 : DiscreteFilter  Numerator=[Ts2/Rth_h_tau]  Denominator=[1 (Ts2/Rth_h_tau)-1]  SampleTime=Ts2
  Gain1 : Gain  Gain=DIODE_344520.Rth_jc1_dou
  Gain2 : Gain  Gain=DIODE_344520.Rth_jc2_dou
  Gain3 : Gain  Gain=DIODE_344520.Rth_jc3_dou
  Gain5 : Gain  Gain=DIODE_344520.Rth_ch_dou
  Gain9 : Gain  Gain=Rth_h
  Out1 : Outport  VectorParamsAs1DForOutWhenUnconnected=off
  wires:
  Discrete Filter9/1 -> Add5/1
  Gain9/1 -> Discrete Filter9/1
  Add3/1 -> Gain2/1, Gain1/1, Gain9/1, Gain5/1, Gain3/1
  Discrete Filter3/1 -> Add4/4
  Gain3/1 -> Discrete Filter3/1
  Discrete Filter5/1 -> Add4/1
  Gain5/1 -> Discrete Filter5/1
  Discrete Filter1/1 -> Add4/2
  Add5/1 -> Out1/1
  Gain1/1 -> Discrete Filter1/1
  Constant/1 -> Add5/3
  In2/1 -> Add3/2
  Add4/1 -> Add5/2
  Discrete Filter2/1 -> Add4/3
  Gain2/1 -> Discrete Filter2/1
  In1/1 -> Add3/1

== system model_sim_CHB5_36_new_temp/Subsystem3/DIODE/DIODE_D1331SH/Subsystem5/Subsystem ==
  In1 : Inport
  Gain44 : Gain  Gain=DIODE.rF
  Gain45 : Gain  Gain=DIODE.VF0
  Math Function9 : Math  Operator=magnitude^2  SignedPower=on  SaturateOnIntegerOverflow=on
  Mean79 : powerlib_meascontrol/Measurements/Mean  Freq=2000  Vinit=0  Ts=Ts1
  RMS9 : powerlib_meascontrol/Measurements/RMS  TrueRMS=on  Freq=2000  RMSInit=0  Ts=Ts1
  Out1 : Outport
  Out2 : Outport  Port=2
  wires:
  Gain45/1 -> Out2/1
  In1/1 -> RMS9/1, Mean79/1
  Math Function9/1 -> Gain44/1
  Mean79/1 -> Gain45/1
  Gain44/1 -> Out1/1
  RMS9/1 -> Math Function9/1

== system model_sim_CHB5_36_new_temp/Subsystem3/DIODE/DIODE_D1331SH/Subsystem5/Subsystem1 ==
  note: 用于判断D1关断时刻，电流为负时，T3开通就意味着D1关断
  In1 : Inport
  In2 : Inport  Port=2
  Abs1 : Abs
  Add : Sum
  Constant1 : Constant  Value=0
  Constant2 : Constant  Value=0
  Gain1 : Gain  Gain=Udc/DIODE.Vdc
  Gain2 : Gain  Gain=DIODE.Err/DIODE.IFQ
  Gain3 : Gain  Gain=1/Ts2
  Gain4 : Gain
  Logical Operator2 : Logic  Operator=NOT  AllPortsSameDT=off  OutDataTypeStr=boolean
  Logical Operator3 : Logic  AllPortsSameDT=off  OutDataTypeStr=boolean
  Logical Operator4 : Logic  AllPortsSameDT=off  OutDataTypeStr=boolean
  Logical Operator5 : Logic  Operator=NOT  AllPortsSameDT=off  OutDataTypeStr=boolean
  Pulse Generator : DiscretePulseGenerator  PulseType=Time based  Period=Ts2  PulseWidth=5
  Saturation : Saturate  UpperLimit=5500  LowerLimit=0
  Saturation1 : Saturate  UpperLimit=100  LowerLimit=0
  Switch2 : Switch  Criteria=u2 > Threshold
  Switch3 : Switch  Criteria=u2 > Threshold
  Switch4 : Switch  Criteria=u2 > Threshold
  Unit Delay{,1..3} (4 alike) : UnitDelay  SampleTime=Ts1  HasFrameUpgradeWarning=on
  Out1 : Outport  VectorParamsAs1DForOutWhenUnconnected=off
  wires:
  Abs1/1 -> Add/1
  Switch2/1 -> Gain1/1
  Gain1/1 -> Abs1/1
  In2/1 -> Logical Operator3/1, Unit Delay/1
  Logical Operator2/1 -> Logical Operator3/2
  Logical Operator3/1 -> Switch2/2
  Constant2/1 -> Switch2/3
  Switch3/1 -> Add/2
  Constant1/1 -> Switch3/1
  Pulse Generator/1 -> Unit Delay3/1, Logical Operator4/1
  Switch4/1 -> Unit Delay2/1, Gain3/1
  Unit Delay2/1 -> Switch4/3
  Unit Delay3/1 -> Logical Operator5/1
  Logical Operator5/1 -> Logical Operator4/2
  Logical Operator4/1 -> Switch4/2, Switch3/2
  Unit Delay1/1 -> Switch3/3, Switch4/1
  Gain3/1 -> Out1/1
  In1/1 -> Gain4/1
  Add/1 -> Unit Delay1/1
  Unit Delay/1 -> Logical Operator2/1
  Gain4/1 -> Saturation/1
  Saturation1/1 -> Switch2/1
  Saturation/1 -> Gain2/1
  Gain2/1 -> Saturation1/1

== system model_sim_CHB5_36_new_temp/Subsystem3/DIODE/DIODE_D1331SH/Subsystem5/Subsystem2 ==
  note: 散热器热阻：水到壳
  note: 器件手册热阻：壳到结
  In1 : Inport
  In2 : Inport  Port=2
  Add3 : Sum
  Add4 : Sum  Inputs=4
  Add5 : Sum  Inputs=+++
  Constant : Constant  Value=temp_init
  Discrete Filter1 : DiscreteFilter  Numerator=[Ts2/DIODE_344520.Rth_jc1_dou_tau]  Denominator=[1 (Ts2/DIODE_344520.Rth_jc1_dou_tau)-1]  SampleTime=Ts2
  Discrete Filter2 : DiscreteFilter  Numerator=[Ts2/DIODE_344520.Rth_jc2_dou_tau]  Denominator=[1 (Ts2/DIODE_344520.Rth_jc2_dou_tau)-1]  SampleTime=Ts2
  Discrete Filter3 : DiscreteFilter  Numerator=[Ts2/DIODE_344520.Rth_jc3_dou_tau]  Denominator=[1 (Ts2/DIODE_344520.Rth_jc3_dou_tau)-1]  SampleTime=Ts2
  Discrete Filter5 : DiscreteFilter  Numerator=[Ts2/DIODE_344520.Rth_ch_dou_tau]  Denominator=[1 (Ts2/DIODE_344520.Rth_ch_dou_tau)-1]  SampleTime=Ts2
  Discrete Filter9 : DiscreteFilter  Numerator=[Ts2/Rth_h_tau]  Denominator=[1 (Ts2/Rth_h_tau)-1]  SampleTime=Ts2
  Gain1 : Gain  Gain=DIODE_344520.Rth_jc1_dou
  Gain2 : Gain  Gain=DIODE_344520.Rth_jc2_dou
  Gain3 : Gain  Gain=DIODE_344520.Rth_jc3_dou
  Gain5 : Gain  Gain=DIODE_344520.Rth_ch_dou
  Gain9 : Gain  Gain=Rth_h
  Out1 : Outport  VectorParamsAs1DForOutWhenUnconnected=off
  wires:
  In1/1 -> Add3/1
  Gain2/1 -> Discrete Filter2/1
  Discrete Filter2/1 -> Add4/3
  Add4/1 -> Add5/2
  In2/1 -> Add3/2
  Constant/1 -> Add5/3
  Gain1/1 -> Discrete Filter1/1
  Add5/1 -> Out1/1
  Discrete Filter1/1 -> Add4/2
  Gain5/1 -> Discrete Filter5/1
  Discrete Filter5/1 -> Add4/1
  Gain3/1 -> Discrete Filter3/1
  Discrete Filter3/1 -> Add4/4
  Add3/1 -> Gain3/1, Gain5/1, Gain9/1, Gain1/1, Gain2/1
  Gain9/1 -> Discrete Filter9/1
  Discrete Filter9/1 -> Add5/1

== system model_sim_CHB5_36_new_temp/Subsystem3/DIODE/DIODE_D1331SH/Subsystem5/Subsystem29 ==
  note: 用于判断D1关断时刻，电流为负时，T3开通就意味着D1关断
  In1 : Inport
  In2 : Inport  Port=2
  Abs1 : Abs
  Add : Sum
  Constant1 : Constant  Value=0
  Constant2 : Constant  Value=0
  Gain1 : Gain  Gain=Udc/DIODE.Vdc
  Gain2 : Gain  Gain=DIODE.Err/DIODE.IFQ
  Gain3 : Gain  Gain=1/Ts2
  Gain4 : Gain
  Logical Operator2 : Logic  Operator=NOT  AllPortsSameDT=off  OutDataTypeStr=boolean
  Logical Operator3 : Logic  AllPortsSameDT=off  OutDataTypeStr=boolean
  Logical Operator4 : Logic  AllPortsSameDT=off  OutDataTypeStr=boolean
  Logical Operator5 : Logic  Operator=NOT  AllPortsSameDT=off  OutDataTypeStr=boolean
  Pulse Generator : DiscretePulseGenerator  PulseType=Time based  Period=Ts2  PulseWidth=5
  Saturation : Saturate  UpperLimit=5500  LowerLimit=0
  Saturation1 : Saturate  UpperLimit=100  LowerLimit=0
  Switch2 : Switch  Criteria=u2 > Threshold
  Switch3 : Switch  Criteria=u2 > Threshold
  Switch4 : Switch  Criteria=u2 > Threshold
  Unit Delay{,1..3} (4 alike) : UnitDelay  SampleTime=Ts1  HasFrameUpgradeWarning=on
  Out1 : Outport  VectorParamsAs1DForOutWhenUnconnected=off
  wires:
  Abs1/1 -> Add/1
  Switch2/1 -> Gain1/1
  Gain1/1 -> Abs1/1
  In2/1 -> Logical Operator3/1, Unit Delay/1
  Logical Operator2/1 -> Logical Operator3/2
  Logical Operator3/1 -> Switch2/2
  Constant2/1 -> Switch2/3
  Switch3/1 -> Add/2
  Constant1/1 -> Switch3/1
  Pulse Generator/1 -> Unit Delay3/1, Logical Operator4/1
  Switch4/1 -> Unit Delay2/1, Gain3/1
  Unit Delay2/1 -> Switch4/3
  Unit Delay3/1 -> Logical Operator5/1
  Logical Operator5/1 -> Logical Operator4/2
  Logical Operator4/1 -> Switch4/2, Switch3/2
  Unit Delay1/1 -> Switch3/3, Switch4/1
  Gain3/1 -> Out1/1
  In1/1 -> Gain4/1
  Add/1 -> Unit Delay1/1
  Unit Delay/1 -> Logical Operator2/1
  Gain4/1 -> Saturation/1
  Saturation1/1 -> Switch2/1
  Saturation/1 -> Gain2/1
  Gain2/1 -> Saturation1/1

== system model_sim_CHB5_36_new_temp/Subsystem3/DIODE/DIODE_D1331SH/Subsystem5/Subsystem4 ==
  In1 : Inport
  Gain44 : Gain  Gain=DIODE.rF
  Gain45 : Gain  Gain=DIODE.VF0
  Math Function9 : Math  Operator=magnitude^2  SignedPower=on  SaturateOnIntegerOverflow=on
  Mean79 : powerlib_meascontrol/Measurements/Mean  Freq=2000  Vinit=0  Ts=Ts1
  RMS9 : powerlib_meascontrol/Measurements/RMS  TrueRMS=on  Freq=2000  RMSInit=0  Ts=Ts1
  Out1 : Outport
  Out2 : Outport  Port=2
  wires:
  Gain45/1 -> Out2/1
  In1/1 -> RMS9/1, Mean79/1
  Math Function9/1 -> Gain44/1
  Mean79/1 -> Gain45/1
  Gain44/1 -> Out1/1
  RMS9/1 -> Math Function9/1

== system model_sim_CHB5_36_new_temp/Subsystem3/DIODE/DIODE_D1331SH/Subsystem5/Subsystem53 ==
  note: 散热器热阻：水到壳
  note: 器件手册热阻：壳到结
  In1 : Inport
  In2 : Inport  Port=2
  Add3 : Sum
  Add4 : Sum  Inputs=4
  Add5 : Sum  Inputs=+++
  Constant : Constant  Value=temp_init
  Discrete Filter1 : DiscreteFilter  Numerator=[Ts2/DIODE_344520.Rth_jc1_dou_tau]  Denominator=[1 (Ts2/DIODE_344520.Rth_jc1_dou_tau)-1]  SampleTime=Ts2
  Discrete Filter2 : DiscreteFilter  Numerator=[Ts2/DIODE_344520.Rth_jc2_dou_tau]  Denominator=[1 (Ts2/DIODE_344520.Rth_jc2_dou_tau)-1]  SampleTime=Ts2
  Discrete Filter3 : DiscreteFilter  Numerator=[Ts2/DIODE_344520.Rth_jc3_dou_tau]  Denominator=[1 (Ts2/DIODE_344520.Rth_jc3_dou_tau)-1]  SampleTime=Ts2
  Discrete Filter5 : DiscreteFilter  Numerator=[Ts2/DIODE_344520.Rth_ch_dou_tau]  Denominator=[1 (Ts2/DIODE_344520.Rth_ch_dou_tau)-1]  SampleTime=Ts2
  Discrete Filter9 : DiscreteFilter  Numerator=[Ts2/Rth_h_tau]  Denominator=[1 (Ts2/Rth_h_tau)-1]  SampleTime=Ts2
  Gain1 : Gain  Gain=DIODE_344520.Rth_jc1_dou
  Gain2 : Gain  Gain=DIODE_344520.Rth_jc2_dou
  Gain3 : Gain  Gain=DIODE_344520.Rth_jc3_dou
  Gain5 : Gain  Gain=DIODE_344520.Rth_ch_dou
  Gain9 : Gain  Gain=Rth_h
  Out1 : Outport  VectorParamsAs1DForOutWhenUnconnected=off
  wires:
  In1/1 -> Add3/1
  Gain2/1 -> Discrete Filter2/1
  Discrete Filter2/1 -> Add4/3
  Add4/1 -> Add5/2
  In2/1 -> Add3/2
  Constant/1 -> Add5/3
  Gain1/1 -> Discrete Filter1/1
  Add5/1 -> Out1/1
  Discrete Filter1/1 -> Add4/2
  Gain5/1 -> Discrete Filter5/1
  Discrete Filter5/1 -> Add4/1
  Gain3/1 -> Discrete Filter3/1
  Discrete Filter3/1 -> Add4/4
  Add3/1 -> Gain3/1, Gain5/1, Gain9/1, Gain1/1, Gain2/1
  Gain9/1 -> Discrete Filter9/1
  Discrete Filter9/1 -> Add5/1

== system model_sim_CHB5_36_new_temp/Subsystem3/IGCT/IGCT_364520_36/MAIN/Subsystem3 ==
  i : Inport
  pwm : Inport  Port=2
  Abs1 : Abs
  Add : Sum
  Constant1 : Constant  Value=0
  Constant2 : Constant  Value=0
  Gain1 : Gain  Gain=Udc/IGCT.Vdc
  Gain2 : Gain  Gain=IGCT.Eon/IGCT.IT*Udc/IGCT.Vdc
  Gain3 : Gain  Gain=1/Ts2
  Gain4 : Gain
  Logical Operator : Logic  AllPortsSameDT=off  OutDataTypeStr=boolean
  Logical Operator1 : Logic  Operator=NOT  AllPortsSameDT=off  OutDataTypeStr=boolean
  Logical Operator2 : Logic  Operator=NOT  AllPortsSameDT=off  OutDataTypeStr=boolean
  Logical Operator3 : Logic  AllPortsSameDT=off  OutDataTypeStr=boolean
  Logical Operator4 : Logic  AllPortsSameDT=off  OutDataTypeStr=boolean
  Logical Operator5 : Logic  Operator=NOT  AllPortsSameDT=off  OutDataTypeStr=boolean
  Polynomial : Polyval  Coefs=IGCT.poly
  Pulse Generator : DiscretePulseGenerator  PulseType=Time based  Period=Ts2  PulseWidth=5
  Switch{1..4} (4 alike) : Switch  Criteria=u2 > Threshold
  Unit Delay{,1..3} (4 alike) : UnitDelay  SampleTime=1e-6  HasFrameUpgradeWarning=on
  PS : Outport  VectorParamsAs1DForOutWhenUnconnected=off
  wires:
  pwm/1 -> Logical Operator2/1, Logical Operator/1, Unit Delay/1
  Logical Operator/1 -> Switch1/2
  Abs1/1 -> Add/1
  Switch2/1 -> Gain1/1
  Switch1/1 -> Abs1/1
  Unit Delay/1 -> Logical Operator3/1, Logical Operator1/1
  Logical Operator1/1 -> Logical Operator/2
  Logical Operator2/1 -> Logical Operator3/2
  Logical Operator3/1 -> Switch2/2
  Constant2/1 -> Switch2/3
  Gain2/1 -> Switch1/1
  Gain1/1 -> Switch1/3
  Switch3/1 -> Add/2
  Constant1/1 -> Switch3/1
  Pulse Generator/1 -> Unit Delay3/1, Logical Operator4/1
  Switch4/1 -> Unit Delay2/1, Gain3/1
  Unit Delay2/1 -> Switch4/3
  Unit Delay3/1 -> Logical Operator5/1
  Logical Operator5/1 -> Logical Operator4/2
  Logical Operator4/1 -> Switch4/2, Switch3/2
  Unit Delay1/1 -> Switch3/3, Switch4/1
  Gain3/1 -> PS/1
  i/1 -> Gain4/1
  Add/1 -> Unit Delay1/1
  Gain4/1 -> Polynomial/1, Gain2/1
  Polynomial/1 -> Switch2/1

== system model_sim_CHB5_36_new_temp/Subsystem3/IGCT/IGCT_364520_36/MAIN/Subsystem31 ==
  note: ch_double
  AVG : Inport
  SW : Inport  Port=2
  Add1 : Sum  Inputs=5
  Add2 : Sum  Inputs=+++
  Add3 : Sum
  Constant1 : Constant  Value=temp_init
  Discrete Filter1 : DiscreteFilter  Numerator=[Ts2/IGCT.Rth_ch_dou_tau]  Denominator=[1 (Ts2/IGCT.Rth_ch_dou_tau)-1]  SampleTime=Ts2
  Discrete Filter2 : DiscreteFilter  Numerator=[Ts2/IGCT.Rth_jc3_dou_tau]  Denominator=[1 (Ts2/IGCT.Rth_jc3_dou_tau)-1]  SampleTime=Ts2
  Discrete Filter3 : DiscreteFilter  Numerator=[Ts2/IGCT.Rth_jc4_dou_tau]  Denominator=[1 (Ts2/IGCT.Rth_jc4_dou_tau)-1]  SampleTime=Ts2
  Discrete Filter5 : DiscreteFilter  Numerator=[Ts2/IGCT.Rth_jc1_dou_tau]  Denominator=[1 (Ts2/IGCT.Rth_jc1_dou_tau)-1]  SampleTime=Ts2
  Discrete Filter6 : DiscreteFilter  Numerator=[Ts2/IGCT.Rth_jc2_dou_tau]  Denominator=[1 (Ts2/IGCT.Rth_jc2_dou_tau)-1]  SampleTime=Ts2
  Discrete Filter9 : DiscreteFilter  Numerator=[Ts2/Rth_h_tau]  Denominator=[1 (Ts2/Rth_h_tau)-1]  SampleTime=Ts2
  Gain1 : Gain  Gain=IGCT.Rth_ch_dou
  Gain5 : Gain  Gain=IGCT.Rth_jc1_dou
  Gain6 : Gain  Gain=IGCT.Rth_jc2_dou
  Gain7 : Gain  Gain=IGCT.Rth_jc3_dou
  Gain8 : Gain  Gain=IGCT.Rth_jc4_dou
  Gain9 : Gain  Gain=Rth_h
  TEMP : Outport  VectorParamsAs1DForOutWhenUnconnected=off
  wires:
  Add3/1 -> Gain9/1, Gain5/1, Gain6/1, Gain7/1, Gain8/1, Gain1/1
  Gain1/1 -> Discrete Filter1/1
  Discrete Filter1/1 -> Add1/5
  Add2/1 -> TEMP/1
  Add1/1 -> Add2/2
  Gain8/1 -> Discrete Filter3/1
  Discrete Filter5/1 -> Add1/1
  Discrete Filter3/1 -> Add1/4
  Discrete Filter2/1 -> Add1/3
  Constant1/1 -> Add2/3
  Gain7/1 -> Discrete Filter2/1
  Discrete Filter6/1 -> Add1/2
  Gain5/1 -> Discrete Filter5/1
  Discrete Filter9/1 -> Add2/1
  Gain9/1 -> Discrete Filter9/1
  Gain6/1 -> Discrete Filter6/1
  SW/1 -> Add3/2
  AVG/1 -> Add3/1

== system model_sim_CHB5_36_new_temp/Subsystem3/IGCT/IGCT_364520_36/MAIN/Subsystem4 ==
  note: ch_double
  AVG : Inport
  SW : Inport  Port=2
  Add1 : Sum  Inputs=5
  Add2 : Sum  Inputs=+++
  Add3 : Sum
  Constant1 : Constant  Value=temp_init
  Discrete Filter1 : DiscreteFilter  Numerator=[Ts2/IGCT.Rth_ch_dou_tau]  Denominator=[1 (Ts2/IGCT.Rth_ch_dou_tau)-1]  SampleTime=Ts2
  Discrete Filter2 : DiscreteFilter  Numerator=[Ts2/IGCT.Rth_jc3_dou_tau]  Denominator=[1 (Ts2/IGCT.Rth_jc3_dou_tau)-1]  SampleTime=Ts2
  Discrete Filter3 : DiscreteFilter  Numerator=[Ts2/IGCT.Rth_jc4_dou_tau]  Denominator=[1 (Ts2/IGCT.Rth_jc4_dou_tau)-1]  SampleTime=Ts2
  Discrete Filter5 : DiscreteFilter  Numerator=[Ts2/IGCT.Rth_jc1_dou_tau]  Denominator=[1 (Ts2/IGCT.Rth_jc1_dou_tau)-1]  SampleTime=Ts2
  Discrete Filter6 : DiscreteFilter  Numerator=[Ts2/IGCT.Rth_jc2_dou_tau]  Denominator=[1 (Ts2/IGCT.Rth_jc2_dou_tau)-1]  SampleTime=Ts2
  Discrete Filter9 : DiscreteFilter  Numerator=[Ts2/Rth_h_tau]  Denominator=[1 (Ts2/Rth_h_tau)-1]  SampleTime=Ts2
  Gain1 : Gain  Gain=IGCT.Rth_ch_dou
  Gain5 : Gain  Gain=IGCT.Rth_jc1_dou
  Gain6 : Gain  Gain=IGCT.Rth_jc2_dou
  Gain7 : Gain  Gain=IGCT.Rth_jc3_dou
  Gain8 : Gain  Gain=IGCT.Rth_jc4_dou
  Gain9 : Gain  Gain=Rth_h
  TEMP : Outport  VectorParamsAs1DForOutWhenUnconnected=off
  wires:
  AVG/1 -> Add3/1
  SW/1 -> Add3/2
  Gain6/1 -> Discrete Filter6/1
  Gain9/1 -> Discrete Filter9/1
  Discrete Filter9/1 -> Add2/1
  Gain5/1 -> Discrete Filter5/1
  Discrete Filter6/1 -> Add1/2
  Gain7/1 -> Discrete Filter2/1
  Constant1/1 -> Add2/3
  Discrete Filter2/1 -> Add1/3
  Discrete Filter3/1 -> Add1/4
  Discrete Filter5/1 -> Add1/1
  Gain8/1 -> Discrete Filter3/1
  Add1/1 -> Add2/2
  Add2/1 -> TEMP/1
  Discrete Filter1/1 -> Add1/5
  Gain1/1 -> Discrete Filter1/1
  Add3/1 -> Gain1/1, Gain8/1, Gain7/1, Gain6/1, Gain5/1, Gain9/1

== system model_sim_CHB5_36_new_temp/Subsystem3/IGCT/IGCT_364520_36/MAIN/Subsystem9 ==
  i : Inport
  pwm : Inport  Port=2
  Abs1 : Abs
  Add : Sum
  Constant1 : Constant  Value=0
  Constant2 : Constant  Value=0
  Gain1 : Gain  Gain=Udc/IGCT.Vdc
  Gain2 : Gain  Gain=IGCT.Eon/IGCT.IT*Udc/IGCT.Vdc
  Gain3 : Gain  Gain=1/Ts2
  Gain4 : Gain
  Logical Operator : Logic  AllPortsSameDT=off  OutDataTypeStr=boolean
  Logical Operator1 : Logic  Operator=NOT  AllPortsSameDT=off  OutDataTypeStr=boolean
  Logical Operator2 : Logic  Operator=NOT  AllPortsSameDT=off  OutDataTypeStr=boolean
  Logical Operator3 : Logic  AllPortsSameDT=off  OutDataTypeStr=boolean
  Logical Operator4 : Logic  AllPortsSameDT=off  OutDataTypeStr=boolean
  Logical Operator5 : Logic  Operator=NOT  AllPortsSameDT=off  OutDataTypeStr=boolean
  Polynomial : Polyval  Coefs=IGCT.poly
  Pulse Generator : DiscretePulseGenerator  PulseType=Time based  Period=Ts2  PulseWidth=5
  Switch{1..4} (4 alike) : Switch  Criteria=u2 > Threshold
  Unit Delay{,1..3} (4 alike) : UnitDelay  SampleTime=1e-6  HasFrameUpgradeWarning=on
  PS : Outport  VectorParamsAs1DForOutWhenUnconnected=off
  wires:
  Polynomial/1 -> Switch2/1
  Gain4/1 -> Gain2/1, Polynomial/1
  Add/1 -> Unit Delay1/1
  i/1 -> Gain4/1
  Gain3/1 -> PS/1
  Unit Delay1/1 -> Switch4/1, Switch3/3
  Logical Operator4/1 -> Switch3/2, Switch4/2
  Logical Operator5/1 -> Logical Operator4/2
  Unit Delay3/1 -> Logical Operator5/1
  Unit Delay2/1 -> Switch4/3
  Switch4/1 -> Gain3/1, Unit Delay2/1
  Pulse Generator/1 -> Logical Operator4/1, Unit Delay3/1
  Constant1/1 -> Switch3/1
  Switch3/1 -> Add/2
  Gain1/1 -> Switch1/3
  Gain2/1 -> Switch1/1
  Constant2/1 -> Switch2/3
  Logical Operator3/1 -> Switch2/2
  Logical Operator2/1 -> Logical Operator3/2
  Logical Operator1/1 -> Logical Operator/2
  Unit Delay/1 -> Logical Operator1/1, Logical Operator3/1
  Switch1/1 -> Abs1/1
  Switch2/1 -> Gain1/1
  Abs1/1 -> Add/1
  Logical Operator/1 -> Switch1/2
  pwm/1 -> Unit Delay/1, Logical Operator/1, Logical Operator2/1

== system model_sim_CHB5_36_new_temp/Subsystem3/IGCT/IGCT_364520_36/MAIN/导通损耗 ==
  i : Inport
  pwm : Inport  Port=2
  Add : Sum
  Constant : Constant  Value=0
  Constant1 : Constant  Value=0
  Gain1 : Gain  Gain=IGCT.rT
  Gain2 : Gain  Gain=IGCT.VT0
  Gain3 : Gain
  Logical Operator : Logic  AllPortsSameDT=off  OutDataTypeStr=boolean
  Math Function : Math  Operator=magnitude^2  SignedPower=on  SaturateOnIntegerOverflow=on
  Relational Operator : RelationalOperator  Operator=>  OutDataTypeStr=boolean  RndMeth=Simplest
  Switch13 : Switch  Criteria=u2 > Threshold
  PD : Outport  VectorParamsAs1DForOutWhenUnconnected=off
  wires:
  Constant1/1 -> Switch13/3
  Switch13/1 -> PD/1
  Logical Operator/1 -> Switch13/2
  pwm/1 -> Logical Operator/2
  Relational Operator/1 -> Logical Operator/1
  Constant/1 -> Relational Operator/2
  Gain3/1 -> Math Function/1, Gain2/1
  Gain1/1 -> Add/1
  i/1 -> Gain3/1, Relational Operator/1
  Math Function/1 -> Gain1/1
  Gain2/1 -> Add/2
  Add/1 -> Switch13/1

== system model_sim_CHB5_36_new_temp/Subsystem3/IGCT/IGCT_364520_36/MAIN/导通损耗1 ==
  i : Inport
  pwm : Inport  Port=2
  Add : Sum
  Constant : Constant  Value=0
  Constant1 : Constant  Value=0
  Gain1 : Gain  Gain=IGCT.rT
  Gain2 : Gain  Gain=IGCT.VT0
  Gain3 : Gain
  Logical Operator : Logic  AllPortsSameDT=off  OutDataTypeStr=boolean
  Math Function : Math  Operator=magnitude^2  SignedPower=on  SaturateOnIntegerOverflow=on
  Relational Operator : RelationalOperator  Operator=>  OutDataTypeStr=boolean  RndMeth=Simplest
  Switch13 : Switch  Criteria=u2 > Threshold
  PD : Outport  VectorParamsAs1DForOutWhenUnconnected=off
  wires:
  Add/1 -> Switch13/1
  Gain2/1 -> Add/2
  Math Function/1 -> Gain1/1
  i/1 -> Relational Operator/1, Gain3/1
  Gain1/1 -> Add/1
  Gain3/1 -> Gain2/1, Math Function/1
  Constant/1 -> Relational Operator/2
  Relational Operator/1 -> Logical Operator/1
  pwm/1 -> Logical Operator/2
  Logical Operator/1 -> Switch13/2
  Switch13/1 -> PD/1
  Constant1/1 -> Switch13/3

== system model_sim_CHB5_36_new_temp/Subsystem3/IGCT/IGCT_364521_36/MAIN/Subsystem3 ==
  i : Inport
  pwm : Inport  Port=2
  Abs1 : Abs
  Add : Sum
  Constant1 : Constant  Value=0
  Constant2 : Constant  Value=0
  Gain1 : Gain  Gain=Udc/IGCT.Vdc
  Gain2 : Gain  Gain=IGCT.Eon/IGCT.IT*Udc/IGCT.Vdc
  Gain3 : Gain  Gain=1/Ts2
  Gain4 : Gain
  Logical Operator : Logic  AllPortsSameDT=off  OutDataTypeStr=boolean
  Logical Operator1 : Logic  Operator=NOT  AllPortsSameDT=off  OutDataTypeStr=boolean
  Logical Operator2 : Logic  Operator=NOT  AllPortsSameDT=off  OutDataTypeStr=boolean
  Logical Operator3 : Logic  AllPortsSameDT=off  OutDataTypeStr=boolean
  Logical Operator4 : Logic  AllPortsSameDT=off  OutDataTypeStr=boolean
  Logical Operator5 : Logic  Operator=NOT  AllPortsSameDT=off  OutDataTypeStr=boolean
  Polynomial : Polyval  Coefs=IGCT.poly
  Pulse Generator : DiscretePulseGenerator  PulseType=Time based  Period=Ts2  PulseWidth=5
  Switch{1..4} (4 alike) : Switch  Criteria=u2 > Threshold
  Unit Delay{,1..3} (4 alike) : UnitDelay  SampleTime=1e-6  HasFrameUpgradeWarning=on
  PS : Outport  VectorParamsAs1DForOutWhenUnconnected=off
  wires:
  Polynomial/1 -> Switch2/1
  Gain4/1 -> Gain2/1, Polynomial/1
  Add/1 -> Unit Delay1/1
  i/1 -> Gain4/1
  Gain3/1 -> PS/1
  Unit Delay1/1 -> Switch4/1, Switch3/3
  Logical Operator4/1 -> Switch3/2, Switch4/2
  Logical Operator5/1 -> Logical Operator4/2
  Unit Delay3/1 -> Logical Operator5/1
  Unit Delay2/1 -> Switch4/3
  Switch4/1 -> Gain3/1, Unit Delay2/1
  Pulse Generator/1 -> Logical Operator4/1, Unit Delay3/1
  Constant1/1 -> Switch3/1
  Switch3/1 -> Add/2
  Gain1/1 -> Switch1/3
  Gain2/1 -> Switch1/1
  Constant2/1 -> Switch2/3
  Logical Operator3/1 -> Switch2/2
  Logical Operator2/1 -> Logical Operator3/2
  Logical Operator1/1 -> Logical Operator/2
  Unit Delay/1 -> Logical Operator1/1, Logical Operator3/1
  Switch1/1 -> Abs1/1
  Switch2/1 -> Gain1/1
  Abs1/1 -> Add/1
  Logical Operator/1 -> Switch1/2
  pwm/1 -> Unit Delay/1, Logical Operator/1, Logical Operator2/1

== system model_sim_CHB5_36_new_temp/Subsystem3/IGCT/IGCT_364521_36/MAIN/Subsystem31 ==
  note: ch_double
  AVG : Inport
  SW : Inport  Port=2
  Add1 : Sum  Inputs=5
  Add2 : Sum  Inputs=+++
  Add3 : Sum
  Constant1 : Constant  Value=temp_init
  Discrete Filter1 : DiscreteFilter  Numerator=[Ts2/IGCT.Rth_ch_dou_tau]  Denominator=[1 (Ts2/IGCT.Rth_ch_dou_tau)-1]  SampleTime=Ts2
  Discrete Filter2 : DiscreteFilter  Numerator=[Ts2/IGCT.Rth_jc3_dou_tau]  Denominator=[1 (Ts2/IGCT.Rth_jc3_dou_tau)-1]  SampleTime=Ts2
  Discrete Filter3 : DiscreteFilter  Numerator=[Ts2/IGCT.Rth_jc4_dou_tau]  Denominator=[1 (Ts2/IGCT.Rth_jc4_dou_tau)-1]  SampleTime=Ts2
  Discrete Filter5 : DiscreteFilter  Numerator=[Ts2/IGCT.Rth_jc1_dou_tau]  Denominator=[1 (Ts2/IGCT.Rth_jc1_dou_tau)-1]  SampleTime=Ts2
  Discrete Filter6 : DiscreteFilter  Numerator=[Ts2/IGCT.Rth_jc2_dou_tau]  Denominator=[1 (Ts2/IGCT.Rth_jc2_dou_tau)-1]  SampleTime=Ts2
  Discrete Filter9 : DiscreteFilter  Numerator=[Ts2/Rth_h_tau]  Denominator=[1 (Ts2/Rth_h_tau)-1]  SampleTime=Ts2
  Gain1 : Gain  Gain=IGCT.Rth_ch_dou
  Gain5 : Gain  Gain=IGCT.Rth_jc1_dou
  Gain6 : Gain  Gain=IGCT.Rth_jc2_dou
  Gain7 : Gain  Gain=IGCT.Rth_jc3_dou
  Gain8 : Gain  Gain=IGCT.Rth_jc4_dou
  Gain9 : Gain  Gain=Rth_h
  TEMP : Outport  VectorParamsAs1DForOutWhenUnconnected=off
  wires:
  AVG/1 -> Add3/1
  SW/1 -> Add3/2
  Gain6/1 -> Discrete Filter6/1
  Gain9/1 -> Discrete Filter9/1
  Discrete Filter9/1 -> Add2/1
  Gain5/1 -> Discrete Filter5/1
  Discrete Filter6/1 -> Add1/2
  Gain7/1 -> Discrete Filter2/1
  Constant1/1 -> Add2/3
  Discrete Filter2/1 -> Add1/3
  Discrete Filter3/1 -> Add1/4
  Discrete Filter5/1 -> Add1/1
  Gain8/1 -> Discrete Filter3/1
  Add1/1 -> Add2/2
  Add2/1 -> TEMP/1
  Discrete Filter1/1 -> Add1/5
  Gain1/1 -> Discrete Filter1/1
  Add3/1 -> Gain1/1, Gain8/1, Gain7/1, Gain6/1, Gain5/1, Gain9/1
